simulink model "TPE1"  (R2019b)
settings: Solver=VariableStepAuto  StartTime=0.0  StopTime=10.0  RelTol=1e-3
settings Model: Creator=luis  LastModifiedBy=luis

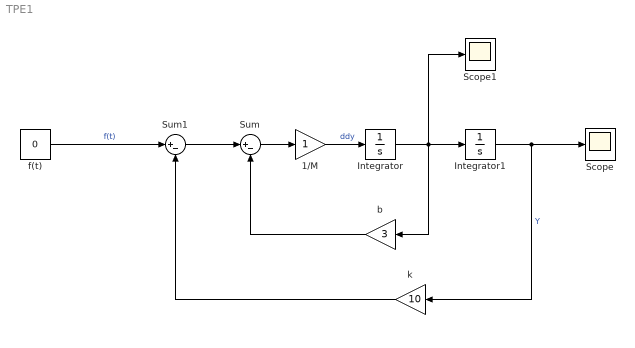
== system TPE1 ==
  "1/M " : Gain
  Integrator : Integrator  InitialCondition=2
  Integrator1 : Integrator  InitialCondition=5
  Scope : Scope
  Scope1 : Scope
  Sum : Sum  Inputs=|+-
  Sum1 : Sum  Inputs=|+-
  b : Gain  Gain=3
  "f(t) " : Constant  Value=0
  k : Gain  Gain=10
  wires:
  Integrator/1 -> Scope1/1, Integrator1/1, b/1
  Integrator1/1 -> Scope/1, k/1  "Y"
  Sum/1 -> "1/M "/1
  "1/M "/1 -> Integrator/1  "ddy"
  Sum1/1 -> Sum/1
  b/1 -> Sum/2
  k/1 -> Sum1/2
  "f(t) "/1 -> Sum1/1  "f(t)"
